simulink model "Ver_0_2"  (R2020a)
settings: Solver=VariableStepAuto  StartTime=0.0  StopTime=10.0  RelTol=1e-3
libraries: simulink x6, dspsigops x3, dsparch4 x3
settings Model: Creator=User  LastModifiedBy=User

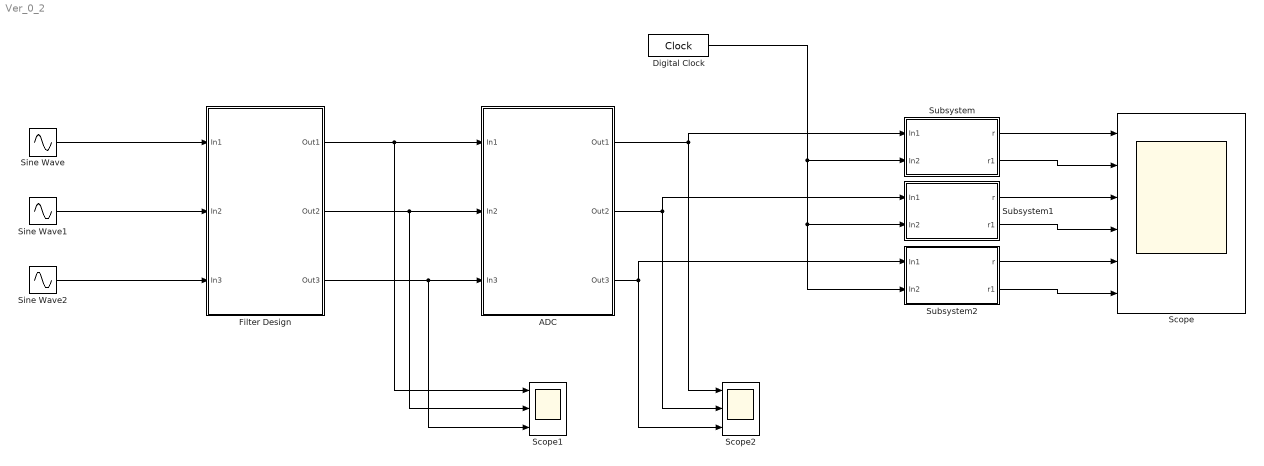
== system Ver_0_2 ==
  ADC : Subsystem
  Digital Clock : DigitalClock
  Filter Design : Subsystem
  Scope : Scope  NumInputPorts=6
  Scope1 : Scope  NumInputPorts=3
  Scope2 : Scope  NumInputPorts=3
  Sine Wave : Sin  SampleTime=0
  Sine Wave1 : Sin  Phase=2*pi/3  SampleTime=0
  Sine Wave2 : Sin  Phase=-2*pi/3  SampleTime=0
  Subsystem : Subsystem
  Subsystem1 : Subsystem
  Subsystem2 : Subsystem
  wires:
  Filter Design/1(Out1) -> Scope1/1, ADC/1(In1)
  Filter Design/2(Out2) -> Scope1/2, ADC/2(In2)
  Filter Design/3(Out3) -> Scope1/3, ADC/3(In3)
  ADC/3(Out3) -> Subsystem2/1(In1), Scope2/3
  ADC/2(Out2) -> Subsystem1/1(In1), Scope2/2
  ADC/1(Out1) -> Subsystem/1(In1), Scope2/1
  Sine Wave/1 -> Filter Design/1(In1)
  Sine Wave1/1 -> Filter Design/2(In2)
  Sine Wave2/1 -> Filter Design/3(In3)
  Subsystem/1(r) -> Scope/1
  Digital Clock/1 -> Subsystem2/2(In2), Subsystem1/2(In2), Subsystem/2(In2)
  Subsystem/2(r1) -> Scope/2
  Subsystem1/1(r) -> Scope/3
  Subsystem1/2(r1) -> Scope/4
  Subsystem2/1(r) -> Scope/5
  Subsystem2/2(r1) -> Scope/6

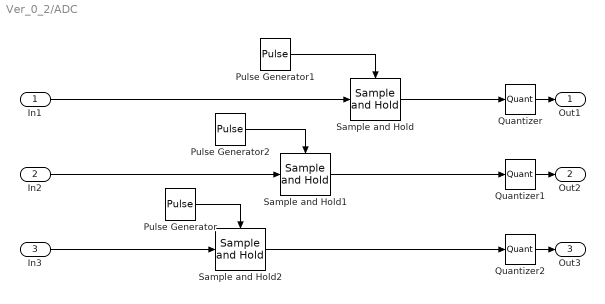
== system Ver_0_2/ADC ==
  In1 : Inport
  In2 : Inport  Port=2
  In3 : Inport  Port=3
  Pulse Generator : DiscretePulseGenerator  PulseType=Time based  Period=0.001  PulseWidth=5
  Pulse Generator1 : DiscretePulseGenerator  PulseType=Time based  Period=0.001  PulseWidth=5
  Pulse Generator2 : DiscretePulseGenerator  PulseType=Time based  Period=0.001  PulseWidth=5
  Quantizer : Quantizer  QuantizationInterval=0.1
  Quantizer1 : Quantizer  QuantizationInterval=0.1
  Quantizer2 : Quantizer  QuantizationInterval=0.1
  Sample and Hold : dspsigops/Sample and Hold  trig=Rising edge  initCond=0  latchinput=off
  Sample and Hold1 : dspsigops/Sample and Hold  trig=Rising edge  initCond=0  latchinput=off
  Sample and Hold2 : dspsigops/Sample and Hold  trig=Rising edge  initCond=0  latchinput=off
  Out1 : Outport
  Out2 : Outport  Port=2
  Out3 : Outport  Port=3
  wires:
  In1/1 -> Sample and Hold/1
  Sample and Hold2/1 -> Quantizer2/1
  Sample and Hold1/1 -> Quantizer1/1
  Pulse Generator1/1 -> Sample and Hold/Trigger
  In2/1 -> Sample and Hold1/1
  Pulse Generator/1 -> Sample and Hold2/Trigger
  Quantizer2/1 -> Out3/1
  Sample and Hold/1 -> Quantizer/1
  Pulse Generator2/1 -> Sample and Hold1/Trigger
  Quantizer/1 -> Out1/1
  Quantizer1/1 -> Out2/1
  In3/1 -> Sample and Hold2/1

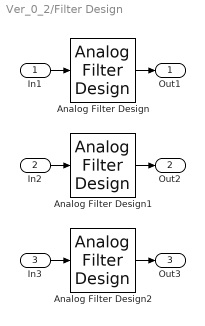
== system Ver_0_2/Filter Design ==
  In1 : Inport
  In2 : Inport  Port=2
  In3 : Inport  Port=3
  Analog Filter Design : dsparch4/Analog Filter Design  method=Butterworth  filttype=Lowpass  N=8  Wlo=30  Whi=80  Rp=2  Rs=40
  Analog Filter Design1 : dsparch4/Analog Filter Design  method=Butterworth  filttype=Lowpass  N=8  Wlo=30  Whi=80  Rp=2  Rs=40
  Analog Filter Design2 : dsparch4/Analog Filter Design  method=Butterworth  filttype=Lowpass  N=8  Wlo=30  Whi=80  Rp=2  Rs=40
  Out1 : Outport
  Out2 : Outport  Port=2
  Out3 : Outport  Port=3
  wires:
  In2/1 -> Analog Filter Design1/1
  Analog Filter Design1/1 -> Out2/1
  In1/1 -> Analog Filter Design/1
  Analog Filter Design2/1 -> Out3/1
  In3/1 -> Analog Filter Design2/1
  Analog Filter Design/1 -> Out1/1

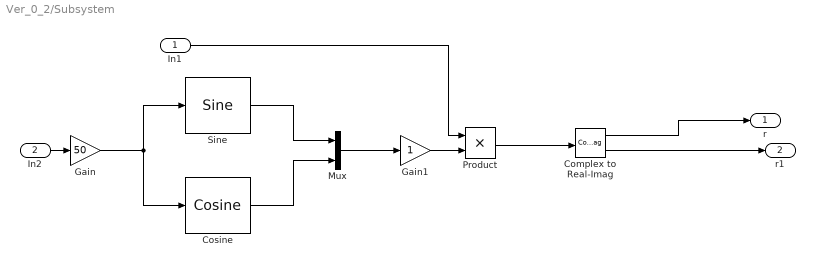
== system Ver_0_2/Subsystem ==
  In1 : Inport
  In2 : Inport  Port=2
  Complex to Real-Imag : ComplexToRealImag
  Cosine : simulink/Lookup Tables/Cosine  Formula=cos(2*pi*u)  NumDataPoints=(2^5)+1  OutputWordLength=16  InternalRulePriority=Speed
      settings: SourceProductBaseCode=SL
  Gain : Gain  Gain=50
  Gain1 : Gain
  Mux : Mux  Inputs=2
  Product : Product
  Sine : simulink/Lookup Tables/Sine  Formula=sin(2*pi*u)  NumDataPoints=(2^5)+1  OutputWordLength=16  InternalRulePriority=Speed
  r : Outport
  r1 : Outport  Port=2
  wires:
  Cosine/1 -> Mux/2
  Mux/1 -> Gain1/1
  Gain/1 -> Sine/1, Cosine/1
  In2/1 -> Gain/1
  Gain1/1 -> Product/2
  Sine/1 -> Mux/1
  In1/1 -> Product/1
  Product/1 -> Complex to Real-Imag/1
  Complex to Real-Imag/1 -> r/1
  Complex to Real-Imag/2 -> r1/1

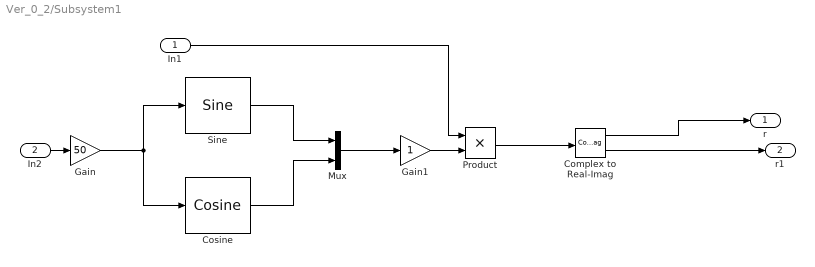
== system Ver_0_2/Subsystem1 ==
  In1 : Inport
  In2 : Inport  Port=2
  Complex to Real-Imag : ComplexToRealImag
  Cosine : simulink/Lookup Tables/Cosine  Formula=cos(2*pi*u)  NumDataPoints=(2^5)+1  OutputWordLength=16  InternalRulePriority=Speed
      settings: SourceProductBaseCode=SL
  Gain : Gain  Gain=50
  Gain1 : Gain
  Mux : Mux  Inputs=2
  Product : Product
  Sine : simulink/Lookup Tables/Sine  Formula=sin(2*pi*u)  NumDataPoints=(2^5)+1  OutputWordLength=16  InternalRulePriority=Speed
  r : Outport
  r1 : Outport  Port=2
  wires:
  Cosine/1 -> Mux/2
  Mux/1 -> Gain1/1
  Gain/1 -> Sine/1, Cosine/1
  In2/1 -> Gain/1
  Gain1/1 -> Product/2
  Sine/1 -> Mux/1
  In1/1 -> Product/1
  Product/1 -> Complex to Real-Imag/1
  Complex to Real-Imag/1 -> r/1
  Complex to Real-Imag/2 -> r1/1

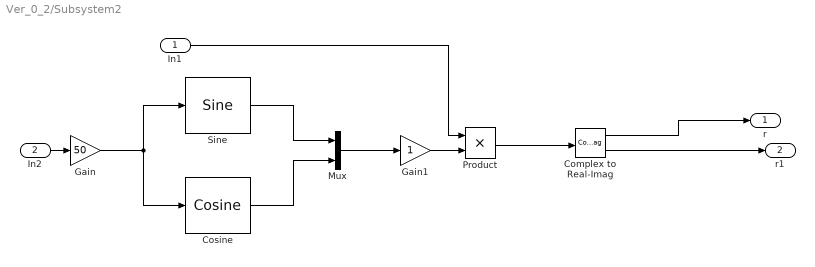
== system Ver_0_2/Subsystem2 ==
  In1 : Inport
  In2 : Inport  Port=2
  Complex to Real-Imag : ComplexToRealImag
  Cosine : simulink/Lookup Tables/Cosine  Formula=cos(2*pi*u)  NumDataPoints=(2^5)+1  OutputWordLength=16  InternalRulePriority=Speed
      settings: SourceProductBaseCode=SL
  Gain : Gain  Gain=50
  Gain1 : Gain
  Mux : Mux  Inputs=2
  Product : Product
  Sine : simulink/Lookup Tables/Sine  Formula=sin(2*pi*u)  NumDataPoints=(2^5)+1  OutputWordLength=16  InternalRulePriority=Speed
  r : Outport
  r1 : Outport  Port=2
  wires:
  Cosine/1 -> Mux/2
  Mux/1 -> Gain1/1
  Gain/1 -> Sine/1, Cosine/1
  In2/1 -> Gain/1
  Gain1/1 -> Product/2
  Sine/1 -> Mux/1
  In1/1 -> Product/1
  Product/1 -> Complex to Real-Imag/1
  Complex to Real-Imag/1 -> r/1
  Complex to Real-Imag/2 -> r1/1
